simulink model "TST_FanSpd_VD"  (R2016b)
settings: Solver=FixedStepDiscrete  StartTime=0.0  StopTime=simTime  FixedStep=sampleTime  RelTol=1e-3
values from neighbouring files (symbols this model uses):
  testCase = 1    [initTST_FanSpd_VD_001.m]    (also in initTST_FanSpd_VD_002.m = 2)
libraries: simulink x17, UnitTest_Lib x14
settings Model: Creator=xinchangran  LastModifiedBy=xinchangran
settings DebuggingCC: SignalRangeChecking=error

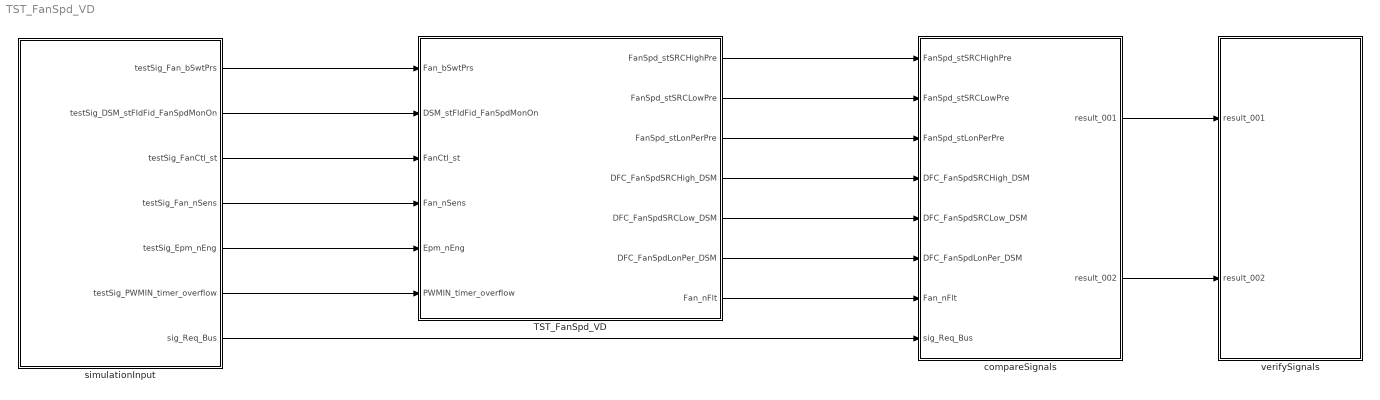
== system TST_FanSpd_VD ==
  TST_FanSpd_VD : Subsystem
  compareSignals : Subsystem
  simulationInput : Subsystem
  verifySignals : Subsystem
  wires:
  simulationInput/1(testSig_Fan_bSwtPrs) -> TST_FanSpd_VD/1(Fan_bSwtPrs)
  simulationInput/2(testSig_DSM_stFIdFid_FanSpdMonOn) -> TST_FanSpd_VD/2(DSM_stFIdFid_FanSpdMonOn)
  simulationInput/3(testSig_FanCtl_st) -> TST_FanSpd_VD/3(FanCtl_st)
  simulationInput/4(testSig_Fan_nSens) -> TST_FanSpd_VD/4(Fan_nSens)
  simulationInput/5(testSig_Epm_nEng) -> TST_FanSpd_VD/5(Epm_nEng)
  simulationInput/6(testSig_PWMIN_timer_overflow) -> TST_FanSpd_VD/6(PWMIN_timer_overflow)
  TST_FanSpd_VD/1(FanSpd_stSRCHighPre) -> compareSignals/1(FanSpd_stSRCHighPre)
  TST_FanSpd_VD/2(FanSpd_stSRCLowPre) -> compareSignals/2(FanSpd_stSRCLowPre)
  TST_FanSpd_VD/3(FanSpd_stLonPerPre) -> compareSignals/3(FanSpd_stLonPerPre)
  TST_FanSpd_VD/4(DFC_FanSpdSRCHigh_DSM) -> compareSignals/4(DFC_FanSpdSRCHigh_DSM)
  TST_FanSpd_VD/5(DFC_FanSpdSRCLow_DSM) -> compareSignals/5(DFC_FanSpdSRCLow_DSM)
  TST_FanSpd_VD/6(DFC_FanSpdLonPer_DSM) -> compareSignals/6(DFC_FanSpdLonPer_DSM)
  TST_FanSpd_VD/7(Fan_nFlt) -> compareSignals/7(Fan_nFlt)
  simulationInput/7(sig_Req_Bus) -> compareSignals/8(sig_Req_Bus)
  compareSignals/1(result_001) -> verifySignals/1(result_001)
  compareSignals/2(result_002) -> verifySignals/2(result_002)

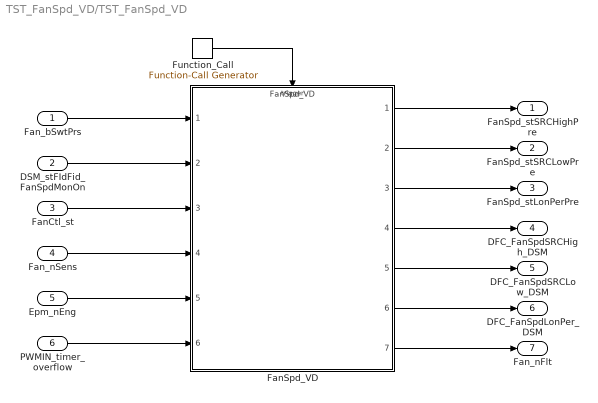
== system TST_FanSpd_VD/TST_FanSpd_VD ==
  Fan_bSwtPrs : Inport
  DSM_stFIdFid_FanSpdMonOn : Inport  Port=2
  FanCtl_st : Inport  Port=3
  Fan_nSens : Inport  Port=4
  Epm_nEng : Inport  Port=5
  PWMIN_timer_overflow : Inport  Port=6
  FanSpd_VD : ModelReference  ModelNameDialog=FanSpd_VD  SimulationMode=Normal  ModelReferenceVersion=1.99  TriggerPortName=function  TriggerPortTriggerType=function-call  TriggerPortStatesWhenEnabling=held
  Function_Call : simulink/Ports & Subsystems/Function-Call Generator  sample_time=sampleTime  numberOfIterations=1
  FanSpd_stSRCHighPre : Outport
  FanSpd_stSRCLowPre : Outport  Port=2
  FanSpd_stLonPerPre : Outport  Port=3
  DFC_FanSpdSRCHigh_DSM : Outport  Port=4
  DFC_FanSpdSRCLow_DSM : Outport  Port=5
  DFC_FanSpdLonPer_DSM : Outport  Port=6
  Fan_nFlt : Outport  Port=7
  wires:
  Function_Call/1 -> FanSpd_VD/Trigger
  Fan_bSwtPrs/1 -> FanSpd_VD/1
  DSM_stFIdFid_FanSpdMonOn/1 -> FanSpd_VD/2
  FanCtl_st/1 -> FanSpd_VD/3
  Fan_nSens/1 -> FanSpd_VD/4
  Epm_nEng/1 -> FanSpd_VD/5
  PWMIN_timer_overflow/1 -> FanSpd_VD/6
  FanSpd_VD/1 -> FanSpd_stSRCHighPre/1
  FanSpd_VD/2 -> FanSpd_stSRCLowPre/1
  FanSpd_VD/3 -> FanSpd_stLonPerPre/1
  FanSpd_VD/4 -> DFC_FanSpdSRCHigh_DSM/1
  FanSpd_VD/5 -> DFC_FanSpdSRCLow_DSM/1
  FanSpd_VD/6 -> DFC_FanSpdLonPer_DSM/1
  FanSpd_VD/7 -> Fan_nFlt/1

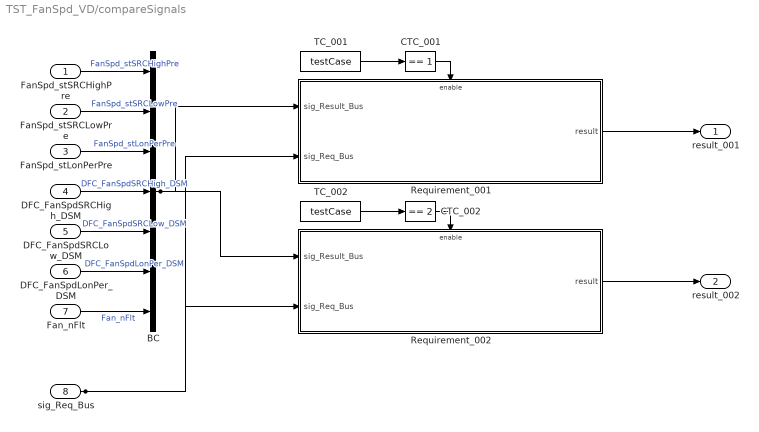
== system TST_FanSpd_VD/compareSignals ==
  FanSpd_stSRCHighPre : Inport
  FanSpd_stSRCLowPre : Inport  Port=2
  FanSpd_stLonPerPre : Inport  Port=3
  DFC_FanSpdSRCHigh_DSM : Inport  Port=4
  DFC_FanSpdSRCLow_DSM : Inport  Port=5
  DFC_FanSpdLonPer_DSM : Inport  Port=6
  Fan_nFlt : Inport  Port=7
  sig_Req_Bus : Inport  Port=8
  BC : BusCreator  Inputs=7
  CTC_001 : simulink/Logic and Bit Operations/Compare To Constant  relop===  const=1  OutDataTypeStr=boolean
  CTC_002 : simulink/Logic and Bit Operations/Compare To Constant  relop===  const=2  OutDataTypeStr=boolean
  Requirement_001 : Subsystem
  Requirement_002 : Subsystem
  TC_001 : Constant  Value=testCase
  TC_002 : Constant  Value=testCase
  result_001 : Outport
  result_002 : Outport  Port=2
  wires:
  FanSpd_stSRCHighPre/1 -> BC/1  "FanSpd_stSRCHighPre"
  FanSpd_stSRCLowPre/1 -> BC/2  "FanSpd_stSRCLowPre"
  FanSpd_stLonPerPre/1 -> BC/3  "FanSpd_stLonPerPre"
  DFC_FanSpdSRCHigh_DSM/1 -> BC/4  "DFC_FanSpdSRCHigh_DSM"
  DFC_FanSpdSRCLow_DSM/1 -> BC/5  "DFC_FanSpdSRCLow_DSM"
  DFC_FanSpdLonPer_DSM/1 -> BC/6  "DFC_FanSpdLonPer_DSM"
  Fan_nFlt/1 -> BC/7  "Fan_nFlt"
  TC_001/1 -> CTC_001/1
  CTC_001/1 -> Requirement_001/Enable
  sig_Req_Bus/1 -> Requirement_001/2(sig_Req_Bus), Requirement_002/2(sig_Req_Bus)
  BC/1 -> Requirement_001/1(sig_Result_Bus), Requirement_002/1(sig_Result_Bus)
  Requirement_001/1(result) -> result_001/1
  TC_002/1 -> CTC_002/1
  CTC_002/1 -> Requirement_002/Enable
  Requirement_002/1(result) -> result_002/1

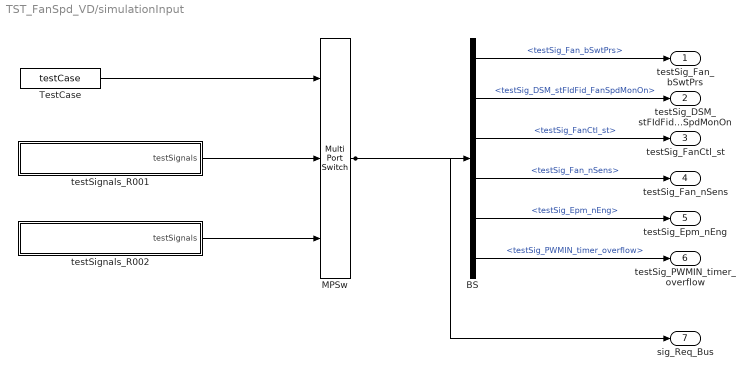
== system TST_FanSpd_VD/simulationInput ==
  BS : BusSelector  OutputSignals=testSig_Fan_bSwtPrs,testSig_DSM_stFIdFid_FanSpdMonOn,testSig_FanCtl_st,testSig_Fan_nSens,testSig_Epm_nEng,testSig_PWMIN_timer_overflow
  MPSw : MultiPortSwitch  Inputs=2  SaturateOnIntegerOverflow=on  InputSameDT=on
  TestCase : Constant  Value=testCase
  testSignals_R001 : Subsystem
  testSignals_R002 : Subsystem
  testSig_Fan_bSwtPrs : Outport
  testSig_DSM_stFIdFid_FanSpdMonOn : Outport  Port=2
  testSig_FanCtl_st : Outport  Port=3
  testSig_Fan_nSens : Outport  Port=4
  testSig_Epm_nEng : Outport  Port=5
  testSig_PWMIN_timer_overflow : Outport  Port=6
  sig_Req_Bus : Outport  Port=7
  wires:
  BS/1 -> testSig_Fan_bSwtPrs/1  "<testSig_Fan_bSwtPrs>"
  BS/2 -> testSig_DSM_stFIdFid_FanSpdMonOn/1  "<testSig_DSM_stFIdFid_FanSpdMonOn>"
  BS/3 -> testSig_FanCtl_st/1  "<testSig_FanCtl_st>"
  BS/4 -> testSig_Fan_nSens/1  "<testSig_Fan_nSens>"
  BS/5 -> testSig_Epm_nEng/1  "<testSig_Epm_nEng>"
  BS/6 -> testSig_PWMIN_timer_overflow/1  "<testSig_PWMIN_timer_overflow>"
  MPSw/1 -> BS/1, sig_Req_Bus/1
  TestCase/1 -> MPSw/1
  testSignals_R001/1(testSignals) -> MPSw/2
  testSignals_R002/1(testSignals) -> MPSw/3

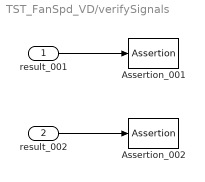
== system TST_FanSpd_VD/verifySignals ==
  result_001 : Inport
  result_002 : Inport  Port=2
  Assertion_001 : Assertion  Enabled=off
  Assertion_002 : Assertion  Enabled=off
  wires:
  result_001/1 -> Assertion_001/1
  result_002/1 -> Assertion_002/1

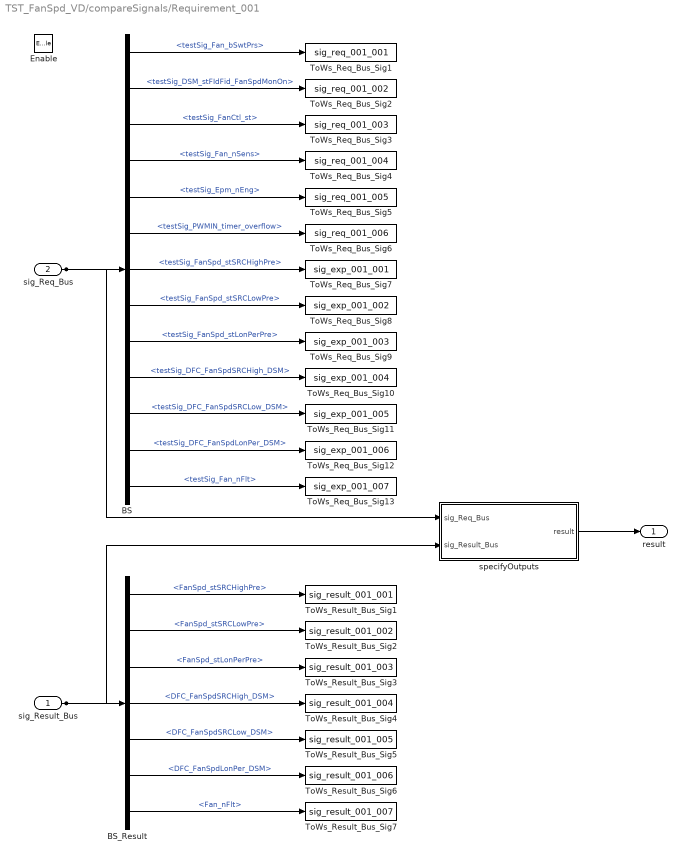
== system TST_FanSpd_VD/compareSignals/Requirement_001 ==
  sig_Result_Bus : Inport
  sig_Req_Bus : Inport  Port=2
  Enable : EnablePort
  BS : BusSelector  OutputSignals=testSig_Fan_bSwtPrs,testSig_DSM_stFIdFid_FanSpdMonOn,testSig_FanCtl_st,testSig_Fan_nSens,testSig_Epm_nEng,testSig_PWMIN_timer_overflow,testSig_FanSpd_stSRCHighPre,testSig_FanSpd_stSRCLowPre,testSig_FanSpd_stLonPerPre,testSig_DFC_FanSpdSRCHigh_DSM,testSig_DFC_FanSpdSRCLow_DSM,testSig_DFC_FanSpdLonPer_DSM,testSig_Fan_nFlt
  BS_Result : BusSelector  OutputSignals=FanSpd_stSRCHighPre,FanSpd_stSRCLowPre,FanSpd_stLonPerPre,DFC_FanSpdSRCHigh_DSM,DFC_FanSpdSRCLow_DSM,DFC_FanSpdLonPer_DSM,Fan_nFlt
  ToWs_Req_Bus_Sig1 : ToWorkspace  VariableName=sig_req_001_001  SaveFormat=Structure With Time
  ToWs_Req_Bus_Sig10 : ToWorkspace  VariableName=sig_exp_001_004  SaveFormat=Structure With Time
  ToWs_Req_Bus_Sig11 : ToWorkspace  VariableName=sig_exp_001_005  SaveFormat=Structure With Time
  ToWs_Req_Bus_Sig12 : ToWorkspace  VariableName=sig_exp_001_006  SaveFormat=Structure With Time
  ToWs_Req_Bus_Sig13 : ToWorkspace  VariableName=sig_exp_001_007  SaveFormat=Structure With Time
  ToWs_Req_Bus_Sig2 : ToWorkspace  VariableName=sig_req_001_002  SaveFormat=Structure With Time
  ToWs_Req_Bus_Sig3 : ToWorkspace  VariableName=sig_req_001_003  SaveFormat=Structure With Time
  ToWs_Req_Bus_Sig4 : ToWorkspace  VariableName=sig_req_001_004  SaveFormat=Structure With Time
  ToWs_Req_Bus_Sig5 : ToWorkspace  VariableName=sig_req_001_005  SaveFormat=Structure With Time
  ToWs_Req_Bus_Sig6 : ToWorkspace  VariableName=sig_req_001_006  SaveFormat=Structure With Time
  ToWs_Req_Bus_Sig7 : ToWorkspace  VariableName=sig_exp_001_001  SaveFormat=Structure With Time
  ToWs_Req_Bus_Sig8 : ToWorkspace  VariableName=sig_exp_001_002  SaveFormat=Structure With Time
  ToWs_Req_Bus_Sig9 : ToWorkspace  VariableName=sig_exp_001_003  SaveFormat=Structure With Time
  ToWs_Result_Bus_Sig1 : ToWorkspace  VariableName=sig_result_001_001  SaveFormat=Structure With Time
  ToWs_Result_Bus_Sig2 : ToWorkspace  VariableName=sig_result_001_002  SaveFormat=Structure With Time
  ToWs_Result_Bus_Sig3 : ToWorkspace  VariableName=sig_result_001_003  SaveFormat=Structure With Time
  ToWs_Result_Bus_Sig4 : ToWorkspace  VariableName=sig_result_001_004  SaveFormat=Structure With Time
  ToWs_Result_Bus_Sig5 : ToWorkspace  VariableName=sig_result_001_005  SaveFormat=Structure With Time
  ToWs_Result_Bus_Sig6 : ToWorkspace  VariableName=sig_result_001_006  SaveFormat=Structure With Time
  ToWs_Result_Bus_Sig7 : ToWorkspace  VariableName=sig_result_001_007  SaveFormat=Structure With Time
  specifyOutputs : Subsystem
  result : Outport
  wires:
  sig_Req_Bus/1 -> BS/1, specifyOutputs/1(sig_Req_Bus)
  BS/1 -> ToWs_Req_Bus_Sig1/1  "<testSig_Fan_bSwtPrs>"
  BS/2 -> ToWs_Req_Bus_Sig2/1  "<testSig_DSM_stFIdFid_FanSpdMonOn>"
  BS/3 -> ToWs_Req_Bus_Sig3/1  "<testSig_FanCtl_st>"
  BS/4 -> ToWs_Req_Bus_Sig4/1  "<testSig_Fan_nSens>"
  BS/5 -> ToWs_Req_Bus_Sig5/1  "<testSig_Epm_nEng>"
  BS/6 -> ToWs_Req_Bus_Sig6/1  "<testSig_PWMIN_timer_overflow>"
  BS/7 -> ToWs_Req_Bus_Sig7/1  "<testSig_FanSpd_stSRCHighPre>"
  BS/8 -> ToWs_Req_Bus_Sig8/1  "<testSig_FanSpd_stSRCLowPre>"
  BS/9 -> ToWs_Req_Bus_Sig9/1  "<testSig_FanSpd_stLonPerPre>"
  BS/10 -> ToWs_Req_Bus_Sig10/1  "<testSig_DFC_FanSpdSRCHigh_DSM>"
  BS/11 -> ToWs_Req_Bus_Sig11/1  "<testSig_DFC_FanSpdSRCLow_DSM>"
  BS/12 -> ToWs_Req_Bus_Sig12/1  "<testSig_DFC_FanSpdLonPer_DSM>"
  BS/13 -> ToWs_Req_Bus_Sig13/1  "<testSig_Fan_nFlt>"
  sig_Result_Bus/1 -> BS_Result/1, specifyOutputs/2(sig_Result_Bus)
  BS_Result/1 -> ToWs_Result_Bus_Sig1/1  "<FanSpd_stSRCHighPre>"
  BS_Result/2 -> ToWs_Result_Bus_Sig2/1  "<FanSpd_stSRCLowPre>"
  BS_Result/3 -> ToWs_Result_Bus_Sig3/1  "<FanSpd_stLonPerPre>"
  BS_Result/4 -> ToWs_Result_Bus_Sig4/1  "<DFC_FanSpdSRCHigh_DSM>"
  BS_Result/5 -> ToWs_Result_Bus_Sig5/1  "<DFC_FanSpdSRCLow_DSM>"
  BS_Result/6 -> ToWs_Result_Bus_Sig6/1  "<DFC_FanSpdLonPer_DSM>"
  BS_Result/7 -> ToWs_Result_Bus_Sig7/1  "<Fan_nFlt>"
  specifyOutputs/1(result) -> result/1

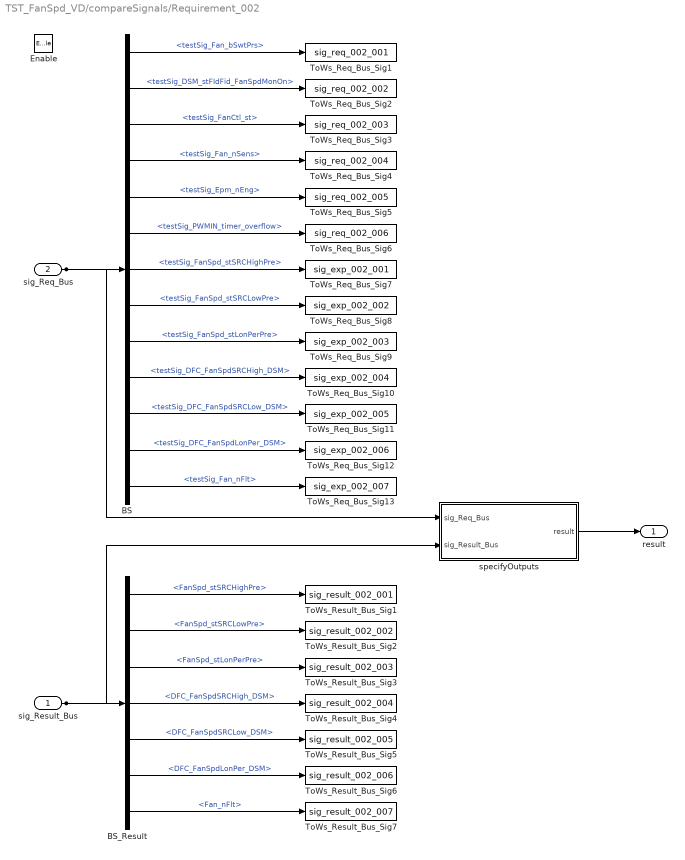
== system TST_FanSpd_VD/compareSignals/Requirement_002 ==
  sig_Result_Bus : Inport
  sig_Req_Bus : Inport  Port=2
  Enable : EnablePort
  BS : BusSelector  OutputSignals=testSig_Fan_bSwtPrs,testSig_DSM_stFIdFid_FanSpdMonOn,testSig_FanCtl_st,testSig_Fan_nSens,testSig_Epm_nEng,testSig_PWMIN_timer_overflow,testSig_FanSpd_stSRCHighPre,testSig_FanSpd_stSRCLowPre,testSig_FanSpd_stLonPerPre,testSig_DFC_FanSpdSRCHigh_DSM,testSig_DFC_FanSpdSRCLow_DSM,testSig_DFC_FanSpdLonPer_DSM,testSig_Fan_nFlt
  BS_Result : BusSelector  OutputSignals=FanSpd_stSRCHighPre,FanSpd_stSRCLowPre,FanSpd_stLonPerPre,DFC_FanSpdSRCHigh_DSM,DFC_FanSpdSRCLow_DSM,DFC_FanSpdLonPer_DSM,Fan_nFlt
  ToWs_Req_Bus_Sig1 : ToWorkspace  VariableName=sig_req_002_001  SaveFormat=Structure With Time
  ToWs_Req_Bus_Sig10 : ToWorkspace  VariableName=sig_exp_002_004  SaveFormat=Structure With Time
  ToWs_Req_Bus_Sig11 : ToWorkspace  VariableName=sig_exp_002_005  SaveFormat=Structure With Time
  ToWs_Req_Bus_Sig12 : ToWorkspace  VariableName=sig_exp_002_006  SaveFormat=Structure With Time
  ToWs_Req_Bus_Sig13 : ToWorkspace  VariableName=sig_exp_002_007  SaveFormat=Structure With Time
  ToWs_Req_Bus_Sig2 : ToWorkspace  VariableName=sig_req_002_002  SaveFormat=Structure With Time
  ToWs_Req_Bus_Sig3 : ToWorkspace  VariableName=sig_req_002_003  SaveFormat=Structure With Time
  ToWs_Req_Bus_Sig4 : ToWorkspace  VariableName=sig_req_002_004  SaveFormat=Structure With Time
  ToWs_Req_Bus_Sig5 : ToWorkspace  VariableName=sig_req_002_005  SaveFormat=Structure With Time
  ToWs_Req_Bus_Sig6 : ToWorkspace  VariableName=sig_req_002_006  SaveFormat=Structure With Time
  ToWs_Req_Bus_Sig7 : ToWorkspace  VariableName=sig_exp_002_001  SaveFormat=Structure With Time
  ToWs_Req_Bus_Sig8 : ToWorkspace  VariableName=sig_exp_002_002  SaveFormat=Structure With Time
  ToWs_Req_Bus_Sig9 : ToWorkspace  VariableName=sig_exp_002_003  SaveFormat=Structure With Time
  ToWs_Result_Bus_Sig1 : ToWorkspace  VariableName=sig_result_002_001  SaveFormat=Structure With Time
  ToWs_Result_Bus_Sig2 : ToWorkspace  VariableName=sig_result_002_002  SaveFormat=Structure With Time
  ToWs_Result_Bus_Sig3 : ToWorkspace  VariableName=sig_result_002_003  SaveFormat=Structure With Time
  ToWs_Result_Bus_Sig4 : ToWorkspace  VariableName=sig_result_002_004  SaveFormat=Structure With Time
  ToWs_Result_Bus_Sig5 : ToWorkspace  VariableName=sig_result_002_005  SaveFormat=Structure With Time
  ToWs_Result_Bus_Sig6 : ToWorkspace  VariableName=sig_result_002_006  SaveFormat=Structure With Time
  ToWs_Result_Bus_Sig7 : ToWorkspace  VariableName=sig_result_002_007  SaveFormat=Structure With Time
  specifyOutputs : Subsystem
  result : Outport
  wires:
  sig_Req_Bus/1 -> BS/1, specifyOutputs/1(sig_Req_Bus)
  BS/1 -> ToWs_Req_Bus_Sig1/1  "<testSig_Fan_bSwtPrs>"
  BS/2 -> ToWs_Req_Bus_Sig2/1  "<testSig_DSM_stFIdFid_FanSpdMonOn>"
  BS/3 -> ToWs_Req_Bus_Sig3/1  "<testSig_FanCtl_st>"
  BS/4 -> ToWs_Req_Bus_Sig4/1  "<testSig_Fan_nSens>"
  BS/5 -> ToWs_Req_Bus_Sig5/1  "<testSig_Epm_nEng>"
  BS/6 -> ToWs_Req_Bus_Sig6/1  "<testSig_PWMIN_timer_overflow>"
  BS/7 -> ToWs_Req_Bus_Sig7/1  "<testSig_FanSpd_stSRCHighPre>"
  BS/8 -> ToWs_Req_Bus_Sig8/1  "<testSig_FanSpd_stSRCLowPre>"
  BS/9 -> ToWs_Req_Bus_Sig9/1  "<testSig_FanSpd_stLonPerPre>"
  BS/10 -> ToWs_Req_Bus_Sig10/1  "<testSig_DFC_FanSpdSRCHigh_DSM>"
  BS/11 -> ToWs_Req_Bus_Sig11/1  "<testSig_DFC_FanSpdSRCLow_DSM>"
  BS/12 -> ToWs_Req_Bus_Sig12/1  "<testSig_DFC_FanSpdLonPer_DSM>"
  BS/13 -> ToWs_Req_Bus_Sig13/1  "<testSig_Fan_nFlt>"
  sig_Result_Bus/1 -> BS_Result/1, specifyOutputs/2(sig_Result_Bus)
  BS_Result/1 -> ToWs_Result_Bus_Sig1/1  "<FanSpd_stSRCHighPre>"
  BS_Result/2 -> ToWs_Result_Bus_Sig2/1  "<FanSpd_stSRCLowPre>"
  BS_Result/3 -> ToWs_Result_Bus_Sig3/1  "<FanSpd_stLonPerPre>"
  BS_Result/4 -> ToWs_Result_Bus_Sig4/1  "<DFC_FanSpdSRCHigh_DSM>"
  BS_Result/5 -> ToWs_Result_Bus_Sig5/1  "<DFC_FanSpdSRCLow_DSM>"
  BS_Result/6 -> ToWs_Result_Bus_Sig6/1  "<DFC_FanSpdLonPer_DSM>"
  BS_Result/7 -> ToWs_Result_Bus_Sig7/1  "<Fan_nFlt>"
  specifyOutputs/1(result) -> result/1

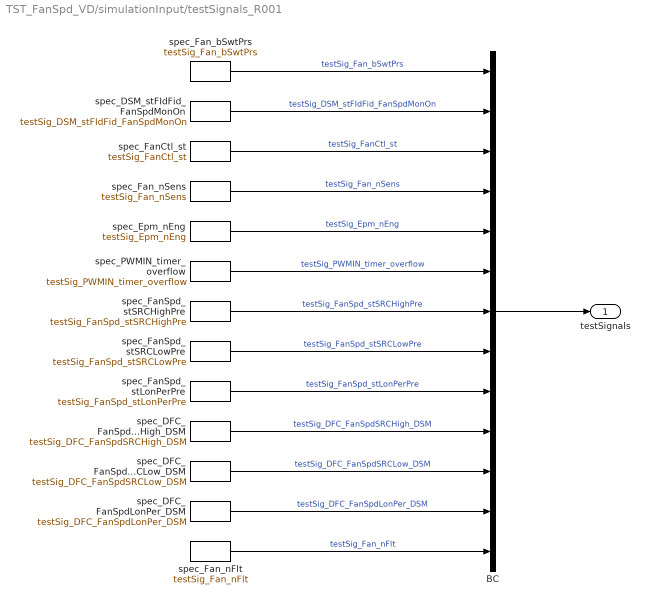
== system TST_FanSpd_VD/simulationInput/testSignals_R001 ==
  BC : BusCreator  Inputs=13
  spec_DFC_FanSpdLonPer_DSM : FromWorkspace  VariableName=testSig_DFC_FanSpdLonPer_DSM  Interpolate=off  OutputAfterFinalValue=Holding final value
  spec_DFC_FanSpdSRCHigh_DSM : FromWorkspace  VariableName=testSig_DFC_FanSpdSRCHigh_DSM  Interpolate=off  OutputAfterFinalValue=Holding final value
  spec_DFC_FanSpdSRCLow_DSM : FromWorkspace  VariableName=testSig_DFC_FanSpdSRCLow_DSM  Interpolate=off  OutputAfterFinalValue=Holding final value
  spec_DSM_stFIdFid_FanSpdMonOn : FromWorkspace  VariableName=testSig_DSM_stFIdFid_FanSpdMonOn  Interpolate=off  OutputAfterFinalValue=Holding final value
  spec_Epm_nEng : FromWorkspace  VariableName=testSig_Epm_nEng  Interpolate=off  OutputAfterFinalValue=Holding final value
  spec_FanCtl_st : FromWorkspace  VariableName=testSig_FanCtl_st  Interpolate=off  OutputAfterFinalValue=Holding final value
  spec_FanSpd_stLonPerPre : FromWorkspace  VariableName=testSig_FanSpd_stLonPerPre  Interpolate=off  OutputAfterFinalValue=Holding final value
  spec_FanSpd_stSRCHighPre : FromWorkspace  VariableName=testSig_FanSpd_stSRCHighPre  Interpolate=off  OutputAfterFinalValue=Holding final value
  spec_FanSpd_stSRCLowPre : FromWorkspace  VariableName=testSig_FanSpd_stSRCLowPre  Interpolate=off  OutputAfterFinalValue=Holding final value
  spec_Fan_bSwtPrs : FromWorkspace  VariableName=testSig_Fan_bSwtPrs  Interpolate=off  OutputAfterFinalValue=Holding final value
  spec_Fan_nFlt : FromWorkspace  VariableName=testSig_Fan_nFlt  Interpolate=off  OutputAfterFinalValue=Holding final value
  spec_Fan_nSens : FromWorkspace  VariableName=testSig_Fan_nSens  Interpolate=off  OutputAfterFinalValue=Holding final value
  spec_PWMIN_timer_overflow : FromWorkspace  VariableName=testSig_PWMIN_timer_overflow  Interpolate=off  OutputAfterFinalValue=Holding final value
  testSignals : Outport
  wires:
  BC/1 -> testSignals/1
  spec_Fan_bSwtPrs/1 -> BC/1  "testSig_Fan_bSwtPrs"
  spec_DSM_stFIdFid_FanSpdMonOn/1 -> BC/2  "testSig_DSM_stFIdFid_FanSpdMonOn"
  spec_FanCtl_st/1 -> BC/3  "testSig_FanCtl_st"
  spec_Fan_nSens/1 -> BC/4  "testSig_Fan_nSens"
  spec_Epm_nEng/1 -> BC/5  "testSig_Epm_nEng"
  spec_PWMIN_timer_overflow/1 -> BC/6  "testSig_PWMIN_timer_overflow"
  spec_FanSpd_stSRCHighPre/1 -> BC/7  "testSig_FanSpd_stSRCHighPre"
  spec_FanSpd_stSRCLowPre/1 -> BC/8  "testSig_FanSpd_stSRCLowPre"
  spec_FanSpd_stLonPerPre/1 -> BC/9  "testSig_FanSpd_stLonPerPre"
  spec_DFC_FanSpdSRCHigh_DSM/1 -> BC/10  "testSig_DFC_FanSpdSRCHigh_DSM"
  spec_DFC_FanSpdSRCLow_DSM/1 -> BC/11  "testSig_DFC_FanSpdSRCLow_DSM"
  spec_DFC_FanSpdLonPer_DSM/1 -> BC/12  "testSig_DFC_FanSpdLonPer_DSM"
  spec_Fan_nFlt/1 -> BC/13  "testSig_Fan_nFlt"

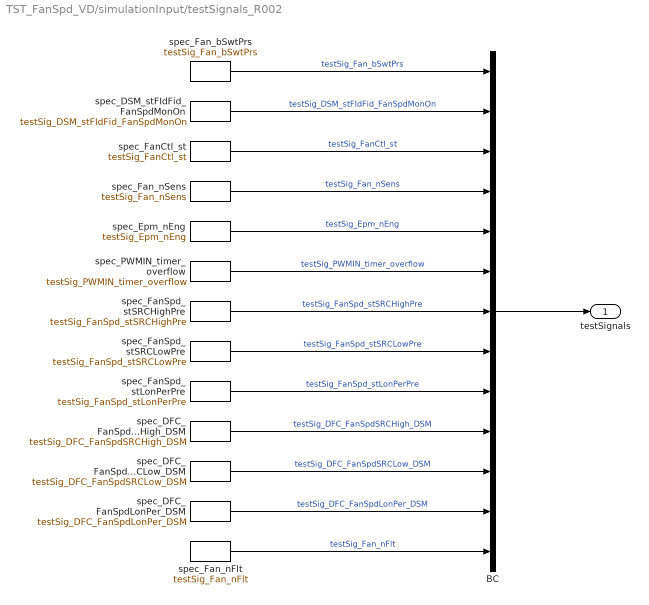
== system TST_FanSpd_VD/simulationInput/testSignals_R002 ==
  BC : BusCreator  Inputs=13
  spec_DFC_FanSpdLonPer_DSM : FromWorkspace  VariableName=testSig_DFC_FanSpdLonPer_DSM  Interpolate=off  OutputAfterFinalValue=Holding final value
  spec_DFC_FanSpdSRCHigh_DSM : FromWorkspace  VariableName=testSig_DFC_FanSpdSRCHigh_DSM  Interpolate=off  OutputAfterFinalValue=Holding final value
  spec_DFC_FanSpdSRCLow_DSM : FromWorkspace  VariableName=testSig_DFC_FanSpdSRCLow_DSM  Interpolate=off  OutputAfterFinalValue=Holding final value
  spec_DSM_stFIdFid_FanSpdMonOn : FromWorkspace  VariableName=testSig_DSM_stFIdFid_FanSpdMonOn  Interpolate=off  OutputAfterFinalValue=Holding final value
  spec_Epm_nEng : FromWorkspace  VariableName=testSig_Epm_nEng  Interpolate=off  OutputAfterFinalValue=Holding final value
  spec_FanCtl_st : FromWorkspace  VariableName=testSig_FanCtl_st  Interpolate=off  OutputAfterFinalValue=Holding final value
  spec_FanSpd_stLonPerPre : FromWorkspace  VariableName=testSig_FanSpd_stLonPerPre  Interpolate=off  OutputAfterFinalValue=Holding final value
  spec_FanSpd_stSRCHighPre : FromWorkspace  VariableName=testSig_FanSpd_stSRCHighPre  Interpolate=off  OutputAfterFinalValue=Holding final value
  spec_FanSpd_stSRCLowPre : FromWorkspace  VariableName=testSig_FanSpd_stSRCLowPre  Interpolate=off  OutputAfterFinalValue=Holding final value
  spec_Fan_bSwtPrs : FromWorkspace  VariableName=testSig_Fan_bSwtPrs  Interpolate=off  OutputAfterFinalValue=Holding final value
  spec_Fan_nFlt : FromWorkspace  VariableName=testSig_Fan_nFlt  Interpolate=off  OutputAfterFinalValue=Holding final value
  spec_Fan_nSens : FromWorkspace  VariableName=testSig_Fan_nSens  Interpolate=off  OutputAfterFinalValue=Holding final value
  spec_PWMIN_timer_overflow : FromWorkspace  VariableName=testSig_PWMIN_timer_overflow  Interpolate=off  OutputAfterFinalValue=Holding final value
  testSignals : Outport
  wires:
  BC/1 -> testSignals/1
  spec_Fan_bSwtPrs/1 -> BC/1  "testSig_Fan_bSwtPrs"
  spec_DSM_stFIdFid_FanSpdMonOn/1 -> BC/2  "testSig_DSM_stFIdFid_FanSpdMonOn"
  spec_FanCtl_st/1 -> BC/3  "testSig_FanCtl_st"
  spec_Fan_nSens/1 -> BC/4  "testSig_Fan_nSens"
  spec_Epm_nEng/1 -> BC/5  "testSig_Epm_nEng"
  spec_PWMIN_timer_overflow/1 -> BC/6  "testSig_PWMIN_timer_overflow"
  spec_FanSpd_stSRCHighPre/1 -> BC/7  "testSig_FanSpd_stSRCHighPre"
  spec_FanSpd_stSRCLowPre/1 -> BC/8  "testSig_FanSpd_stSRCLowPre"
  spec_FanSpd_stLonPerPre/1 -> BC/9  "testSig_FanSpd_stLonPerPre"
  spec_DFC_FanSpdSRCHigh_DSM/1 -> BC/10  "testSig_DFC_FanSpdSRCHigh_DSM"
  spec_DFC_FanSpdSRCLow_DSM/1 -> BC/11  "testSig_DFC_FanSpdSRCLow_DSM"
  spec_DFC_FanSpdLonPer_DSM/1 -> BC/12  "testSig_DFC_FanSpdLonPer_DSM"
  spec_Fan_nFlt/1 -> BC/13  "testSig_Fan_nFlt"

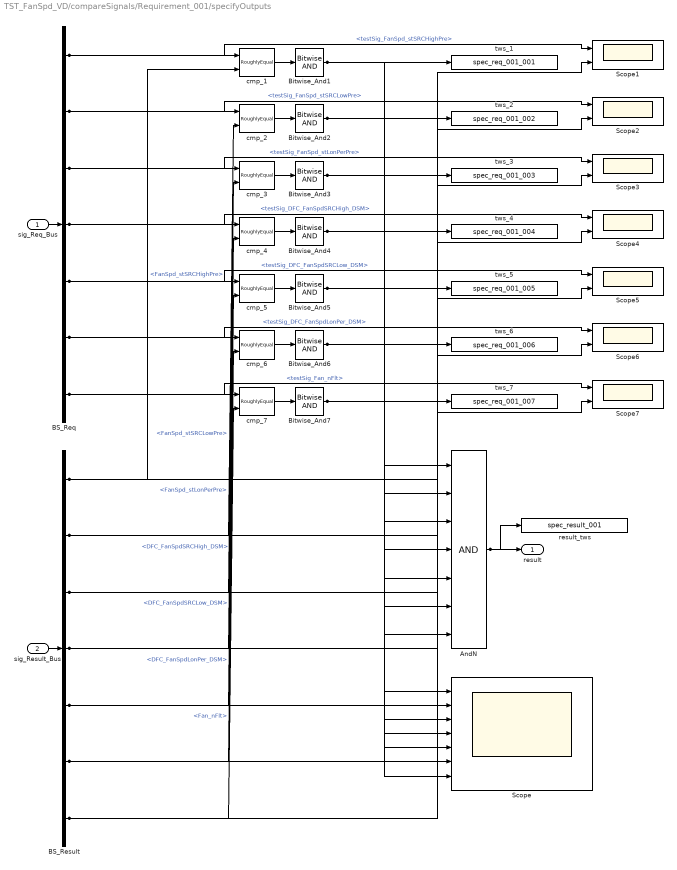
== system TST_FanSpd_VD/compareSignals/Requirement_001/specifyOutputs ==
  sig_Req_Bus : Inport
  sig_Result_Bus : Inport  Port=2
  AndN : Logic  Inputs=7
  BS_Req : BusSelector  OutputSignals=testSig_FanSpd_stSRCHighPre,testSig_FanSpd_stSRCLowPre,testSig_FanSpd_stLonPerPre,testSig_DFC_FanSpdSRCHigh_DSM,testSig_DFC_FanSpdSRCLow_DSM,testSig_DFC_FanSpdLonPer_DSM,testSig_Fan_nFlt
  BS_Result : BusSelector  OutputSignals=FanSpd_stSRCHighPre,FanSpd_stSRCLowPre,FanSpd_stLonPerPre,DFC_FanSpdSRCHigh_DSM,DFC_FanSpdSRCLow_DSM,DFC_FanSpdLonPer_DSM,Fan_nFlt
  Bitwise_And{1..7} (7 alike) : simulink/Logic and Bit Operations/Bitwise Operator  logicop=AND  UseBitMask=off  BitMask=bin2dec('11011001')  BitMaskRealWorld=Stored Integer
  Scope : Scope  NumInputPorts=7
  Scope{1..7} (7 alike) : Scope  NumInputPorts=2
  cmp_{1..7} (7 alike) : UnitTest_Lib/RoughlyEqual  slope=0.1
  result_tws : ToWorkspace  VariableName=spec_result_001
  tws_1 : ToWorkspace  VariableName=spec_req_001_001
  tws_2 : ToWorkspace  VariableName=spec_req_001_002
  tws_3 : ToWorkspace  VariableName=spec_req_001_003
  tws_4 : ToWorkspace  VariableName=spec_req_001_004
  tws_5 : ToWorkspace  VariableName=spec_req_001_005
  tws_6 : ToWorkspace  VariableName=spec_req_001_006
  tws_7 : ToWorkspace  VariableName=spec_req_001_007
  result : Outport
  wires:
  sig_Req_Bus/1 -> BS_Req/1
  sig_Result_Bus/1 -> BS_Result/1
  AndN/1 -> result/1, result_tws/1
  BS_Req/1 -> cmp_1/1, Scope1/1  "<testSig_FanSpd_stSRCHighPre>"
  BS_Result/1 -> cmp_1/2, Scope1/2  "<FanSpd_stSRCHighPre>"
  cmp_1/1 -> Bitwise_And1/1
  Bitwise_And1/1 -> tws_1/1, AndN/1, Scope/1
  BS_Req/2 -> cmp_2/1, Scope2/1  "<testSig_FanSpd_stSRCLowPre>"
  BS_Result/2 -> cmp_2/2, Scope2/2  "<FanSpd_stSRCLowPre>"
  cmp_2/1 -> Bitwise_And2/1
  Bitwise_And2/1 -> tws_2/1, AndN/2, Scope/2
  BS_Req/3 -> cmp_3/1, Scope3/1  "<testSig_FanSpd_stLonPerPre>"
  BS_Result/3 -> cmp_3/2, Scope3/2  "<FanSpd_stLonPerPre>"
  cmp_3/1 -> Bitwise_And3/1
  Bitwise_And3/1 -> tws_3/1, AndN/3, Scope/3
  BS_Req/4 -> cmp_4/1, Scope4/1  "<testSig_DFC_FanSpdSRCHigh_DSM>"
  BS_Result/4 -> cmp_4/2, Scope4/2  "<DFC_FanSpdSRCHigh_DSM>"
  cmp_4/1 -> Bitwise_And4/1
  Bitwise_And4/1 -> tws_4/1, AndN/4, Scope/4
  BS_Req/5 -> cmp_5/1, Scope5/1  "<testSig_DFC_FanSpdSRCLow_DSM>"
  BS_Result/5 -> cmp_5/2, Scope5/2  "<DFC_FanSpdSRCLow_DSM>"
  cmp_5/1 -> Bitwise_And5/1
  Bitwise_And5/1 -> tws_5/1, AndN/5, Scope/5
  BS_Req/6 -> cmp_6/1, Scope6/1  "<testSig_DFC_FanSpdLonPer_DSM>"
  BS_Result/6 -> cmp_6/2, Scope6/2  "<DFC_FanSpdLonPer_DSM>"
  cmp_6/1 -> Bitwise_And6/1
  Bitwise_And6/1 -> tws_6/1, AndN/6, Scope/6
  BS_Req/7 -> cmp_7/1, Scope7/1  "<testSig_Fan_nFlt>"
  BS_Result/7 -> cmp_7/2, Scope7/2  "<Fan_nFlt>"
  cmp_7/1 -> Bitwise_And7/1
  Bitwise_And7/1 -> tws_7/1, AndN/7, Scope/7

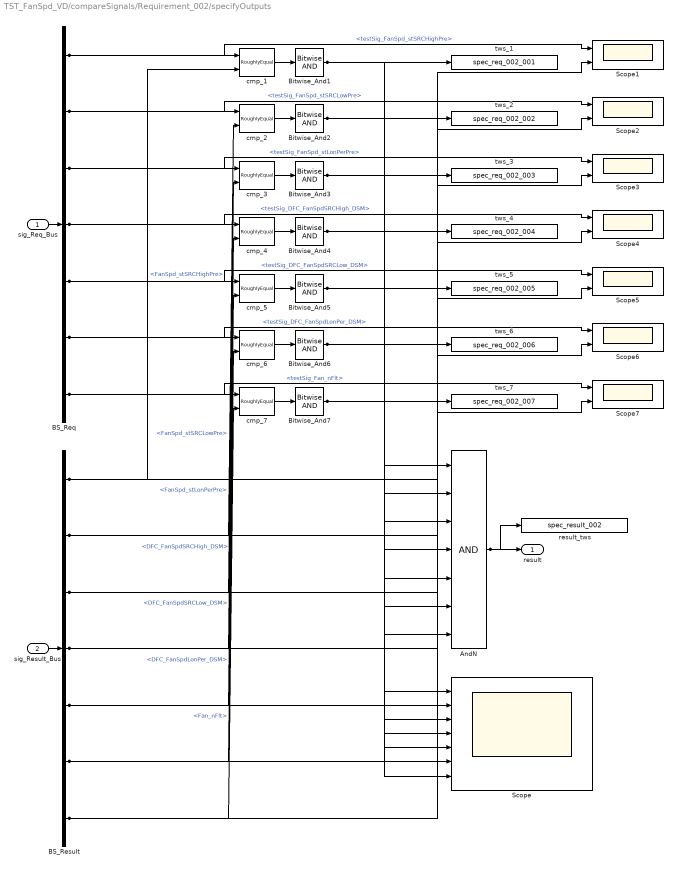
== system TST_FanSpd_VD/compareSignals/Requirement_002/specifyOutputs ==
  sig_Req_Bus : Inport
  sig_Result_Bus : Inport  Port=2
  AndN : Logic  Inputs=7
  BS_Req : BusSelector  OutputSignals=testSig_FanSpd_stSRCHighPre,testSig_FanSpd_stSRCLowPre,testSig_FanSpd_stLonPerPre,testSig_DFC_FanSpdSRCHigh_DSM,testSig_DFC_FanSpdSRCLow_DSM,testSig_DFC_FanSpdLonPer_DSM,testSig_Fan_nFlt
  BS_Result : BusSelector  OutputSignals=FanSpd_stSRCHighPre,FanSpd_stSRCLowPre,FanSpd_stLonPerPre,DFC_FanSpdSRCHigh_DSM,DFC_FanSpdSRCLow_DSM,DFC_FanSpdLonPer_DSM,Fan_nFlt
  Bitwise_And{1..7} (7 alike) : simulink/Logic and Bit Operations/Bitwise Operator  logicop=AND  UseBitMask=off  BitMask=bin2dec('11011001')  BitMaskRealWorld=Stored Integer
  Scope : Scope  NumInputPorts=7
  Scope{1..7} (7 alike) : Scope  NumInputPorts=2
  cmp_{1..7} (7 alike) : UnitTest_Lib/RoughlyEqual  slope=0.1
  result_tws : ToWorkspace  VariableName=spec_result_002
  tws_1 : ToWorkspace  VariableName=spec_req_002_001
  tws_2 : ToWorkspace  VariableName=spec_req_002_002
  tws_3 : ToWorkspace  VariableName=spec_req_002_003
  tws_4 : ToWorkspace  VariableName=spec_req_002_004
  tws_5 : ToWorkspace  VariableName=spec_req_002_005
  tws_6 : ToWorkspace  VariableName=spec_req_002_006
  tws_7 : ToWorkspace  VariableName=spec_req_002_007
  result : Outport
  wires:
  sig_Req_Bus/1 -> BS_Req/1
  sig_Result_Bus/1 -> BS_Result/1
  AndN/1 -> result/1, result_tws/1
  BS_Req/1 -> cmp_1/1, Scope1/1  "<testSig_FanSpd_stSRCHighPre>"
  BS_Result/1 -> cmp_1/2, Scope1/2  "<FanSpd_stSRCHighPre>"
  cmp_1/1 -> Bitwise_And1/1
  Bitwise_And1/1 -> tws_1/1, AndN/1, Scope/1
  BS_Req/2 -> cmp_2/1, Scope2/1  "<testSig_FanSpd_stSRCLowPre>"
  BS_Result/2 -> cmp_2/2, Scope2/2  "<FanSpd_stSRCLowPre>"
  cmp_2/1 -> Bitwise_And2/1
  Bitwise_And2/1 -> tws_2/1, AndN/2, Scope/2
  BS_Req/3 -> cmp_3/1, Scope3/1  "<testSig_FanSpd_stLonPerPre>"
  BS_Result/3 -> cmp_3/2, Scope3/2  "<FanSpd_stLonPerPre>"
  cmp_3/1 -> Bitwise_And3/1
  Bitwise_And3/1 -> tws_3/1, AndN/3, Scope/3
  BS_Req/4 -> cmp_4/1, Scope4/1  "<testSig_DFC_FanSpdSRCHigh_DSM>"
  BS_Result/4 -> cmp_4/2, Scope4/2  "<DFC_FanSpdSRCHigh_DSM>"
  cmp_4/1 -> Bitwise_And4/1
  Bitwise_And4/1 -> tws_4/1, AndN/4, Scope/4
  BS_Req/5 -> cmp_5/1, Scope5/1  "<testSig_DFC_FanSpdSRCLow_DSM>"
  BS_Result/5 -> cmp_5/2, Scope5/2  "<DFC_FanSpdSRCLow_DSM>"
  cmp_5/1 -> Bitwise_And5/1
  Bitwise_And5/1 -> tws_5/1, AndN/5, Scope/5
  BS_Req/6 -> cmp_6/1, Scope6/1  "<testSig_DFC_FanSpdLonPer_DSM>"
  BS_Result/6 -> cmp_6/2, Scope6/2  "<DFC_FanSpdLonPer_DSM>"
  cmp_6/1 -> Bitwise_And6/1
  Bitwise_And6/1 -> tws_6/1, AndN/6, Scope/6
  BS_Req/7 -> cmp_7/1, Scope7/1  "<testSig_Fan_nFlt>"
  BS_Result/7 -> cmp_7/2, Scope7/2  "<Fan_nFlt>"
  cmp_7/1 -> Bitwise_And7/1
  Bitwise_And7/1 -> tws_7/1, AndN/7, Scope/7
